simulink model "vehicle_progetto_v1"  (R2022a)
settings: Solver=ode45  StartTime=0.0  StopTime=200.0  MinStep=1e-60  RelTol=1e-3
values from neighbouring files (symbols this model uses):
  a = 2    [vehicle_parameters.m]    (also in vehicle_parameters_v1.m = 1.3; vehicle_parameters_v1_sospensioni.m = 1.3)
  alpha = atan(w/(2*b))    [vehicle_parameters.m]    (also in vehicle_parameters_v1.m; vehicle_parameters_v1_sospensioni.m)
  b = 2.5    [vehicle_parameters.m]    (also in vehicle_parameters_v1.m = 1.8; vehicle_parameters_v1_sospensioni.m = 1.8)
  ca = 0.5    [vehicle_parameters.m]    (also in vehicle_parameters_v1.m; vehicle_parameters_v1_sospensioni.m)
  cs = sqrt(2*ks*M)    [vehicle_parameters.m]    (also in vehicle_parameters_v1.m; vehicle_parameters_v1_sospensioni.m)
  h_gc = 0.15    [vehicle_parameters.m]    (also in vehicle_parameters_v1.m; vehicle_parameters_v1_sospensioni.m = 0.35)
  J_motore = 0.3    [vehicle_parameters_v1.m]    (also in vehicle_parameters_v1_sospensioni.m)
  J_wheel = 0.4    [vehicle_parameters_v1.m]    (also in vehicle_parameters_v1_sospensioni.m)
  Jx = 300    [vehicle_parameters.m]    (also in vehicle_parameters_v1.m; vehicle_parameters_v1_sospensioni.m)
  Jy = 500    [vehicle_parameters.m]    (also in vehicle_parameters_v1.m; vehicle_parameters_v1_sospensioni.m)
  Jz = 600    [vehicle_parameters.m]    (also in vehicle_parameters_v1.m; vehicle_parameters_v1_sospensioni.m)
  K_elettrica_motore = 0.1    [vehicle_parameters_v1.m]    (also in vehicle_parameters_v1_sospensioni.m)
  K_f_motore = 1    [vehicle_parameters_v1.m]    (also in vehicle_parameters_v1_sospensioni.m)
  K_motore = 1    [vehicle_parameters_v1.m]    (also in vehicle_parameters_v1_sospensioni.m)
  k_r = 1e4    (= 10000)    [vehicle_parameters.m]    (also in vehicle_parameters_v1.m = 2000000; vehicle_parameters_v1_sospensioni.m = 2000000)
  k_tu = 1.5e5    (= 150000)    [vehicle_parameters.m]    (also in vehicle_parameters_v1.m = 1500000; vehicle_parameters_v1_sospensioni.m = 1500000)
  k_tv = 4e4    (= 40000)    [vehicle_parameters.m]    (also in vehicle_parameters_v1.m = 400000; vehicle_parameters_v1_sospensioni.m = 400000)
  ks = 40000    [vehicle_parameters.m]    (also in vehicle_parameters_v1.m; vehicle_parameters_v1_sospensioni.m = 9.75)
  L = sqrt(a^2+w^2 /4)    [vehicle_parameters.m]    (also in vehicle_parameters_v1.m; vehicle_parameters_v1_sospensioni.m)
  L_motore = 0.001100    (= 0.0011)    [vehicle_parameters_v1.m]    (also in vehicle_parameters_v1_sospensioni.m)
  M = 1000    [vehicle_parameters.m]    (also in vehicle_parameters_v1.m; vehicle_parameters_v1_sospensioni.m = 1500)
  mu_dyn = 0.4    [vehicle_parameters.m]    (also in vehicle_parameters_v1.m = 0.2; vehicle_parameters_v1_sospensioni.m = 0.2)
  mu_st = 0.8    [vehicle_parameters.m]    (also in vehicle_parameters_v1.m; vehicle_parameters_v1_sospensioni.m)
  r = 0.2    [vehicle_parameters.m]    (also in vehicle_parameters_v1.m = 0.3; vehicle_parameters_v1_sospensioni.m = 0.3)
  R = sqrt(b^2+w^2 /4)    [vehicle_parameters.m]    (also in vehicle_parameters_v1.m; vehicle_parameters_v1_sospensioni.m)
  R_motore = 0.210    (= 0.21)    [vehicle_parameters_v1.m]    (also in vehicle_parameters_v1_sospensioni.m)
  theta = atan(w/(2*a))    [vehicle_parameters.m]    (also in vehicle_parameters_v1.m; vehicle_parameters_v1_sospensioni.m)
  w = 1.6    [vehicle_parameters.m]    (also in vehicle_parameters_v1.m; vehicle_parameters_v1_sospensioni.m)
libraries: simulink x4, slpidlib x1
settings Model: Creator=jackrip  LastModifiedBy=jackrip

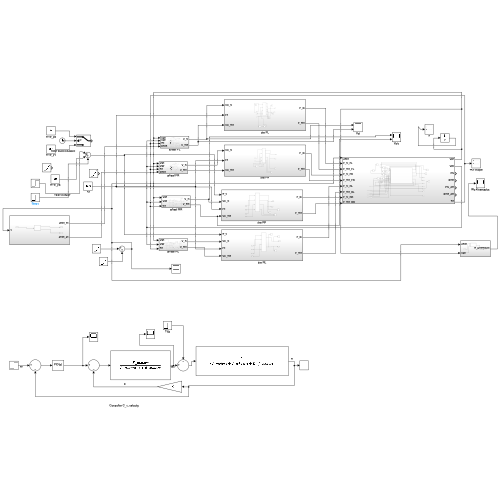
[thumbnail: Simulink's stored preview of the top-level diagram]
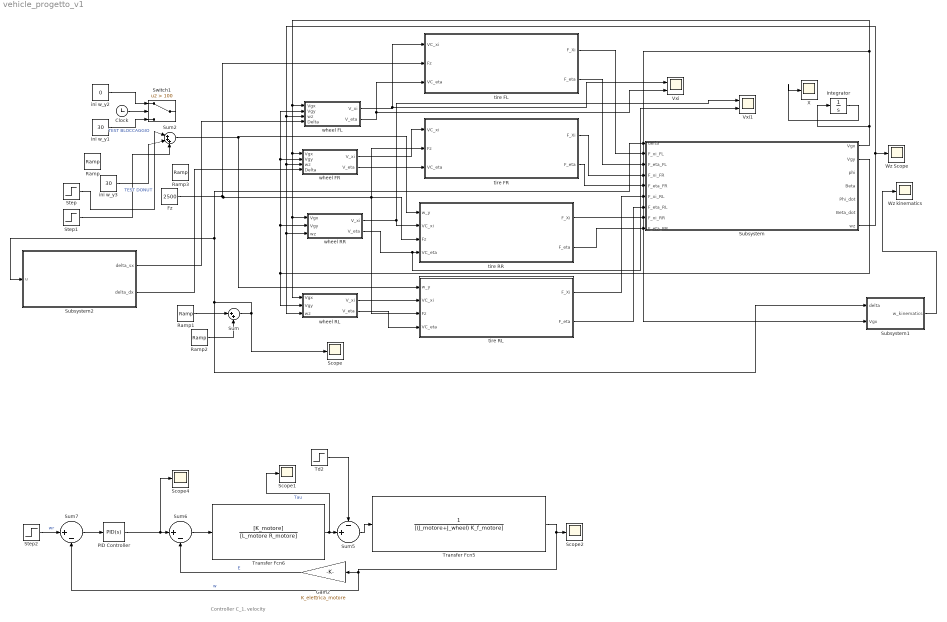
== system vehicle_progetto_v1 ==
  note: Controller C_1, velocity
  " Fz" : Constant  Value=2500
  Clock : Clock
  Gain2 : Gain  Gain=K_elettrica_motore
  Integrator : Integrator
  PID Controller : slpidlib/PID Controller  Controller=PID  Form=Parallel  TimeDomain=Continuous-time  UseExternalTs=off  SampleTime=-1  IntegratorMethod=Forward Euler  FilterMethod=Forward Euler  ControllerParametersSource=internal  P=5  I=1  UseKiTs=off  D=0  N=100  UseFilter=on  TunerSelectOption=Transfer Function Based (PID Tuner App)  InitialConditionSource=internal  InitialConditionForIntegrator=0  InitialConditionForFilter=0  DifferentiatorICPrevScaledInput=0  ExternalReset=none  TrackingMode=off  Kt=1  LimitOutput=off  SatLimitsSource=internal  UpperSaturationLimit=inf  LowerSaturationLimit=-inf  LinearizeAsGain=on  AntiWindupMode=none  Kb=1  POutMin=[]  POutMax=[]  IOutMin=[]  IOutMax=[]  DOutMin=[]  DOutMax=[]  NOutMin=[]  NOutMax=[]  SumOutMin=[]  SumOutMax=[]  SaturationOutMin=[]  SaturationOutMax=[]  PParamMin=[]  PParamMax=[]  IParamMin=[]  IParamMax=[]  DParamMin=[]  DParamMax=[]  NParamMin=[]  NParamMax=[]  KbParamMin=[]  KbParamMax=[]  KtParamMin=[]  KtParamMax=[]  KbOutMin=[]  KbOutMax=[]  KtOutMin=[]  KtOutMax=[]  IntegratorOutMin=[]  IntegratorOutMax=[]  FilterOutMin=[]  FilterOutMax=[]  SumI1OutMin=[]  SumI1OutMax=[]  SumI2OutMin=[]  SumI2OutMax=[]  SumI3OutMin=[]  SumI3OutMax=[]  SumI4OutMin=[]  SumI4OutMax=[]  SumDOutMin=[]  SumDOutMax=[]  DifferentiatorOutMin=[]  DifferentiatorOutMax=[]  FilterDiffOutCoefMin=[]  FilterDiffOutCoefMax=[]  ReciprocalOutMin=[]  ReciprocalOutMax=[]  SumDenOutMin=[]  SumDenOutMax=[]  SumNumOutMin=[]  SumNumOutMax=[]  DivideOutMin=[]  DivideOutMax=[]  UdiffTsProdOutMin=[]  UdiffTsProdOutMax=[]  NTsProdOutMin=[]  NTsProdOutMax=[]  UintegralTsProdOutMin=[]  UintegralTsProdOutMax=[]  UngainTsProdOutMin=[]  UngainTsProdOutMax=[]  IntegratorContinuousStateAttributes=''  IntegratorStateMustResolveToSignalObject=off  IntegratorRTWStateStorageClass=Auto  FilterContinuousStateAttributes=''  FilterStateMustResolveToSignalObject=off  FilterRTWStateStorageClass=Auto  ParallelPVariant=InternalParameters  IdealPVariant=Disabled  IVariant=InternalParameters  DVariant=InternalParameters  IntegratorVariant=Continuous  SatVariant=Disabled  AWVariant=Passthrough  PCopyVariant=Disabled  TRVariant=Disabled  FdbkBlocksVariant=Forward  IdealPFdbkVariant=Disabled  SatFdbkVariant=Disabled  DerivativeFilterVariant=ContFilter  NVariant=InternalParameters  NCopyVariant=Disabled  FilterICVariant=InternalICsFilter  IntegratorICVariant=InternalICs  ExternalResetVariant=Disabled  TRSumVariant=Passthrough  SumFdbkVariant=Disabled  SumVariant=Sum_PID  TsampFilterVariant=InternalTs  TsampNgainVariant=Passthrough  TsampIntegralVariant=Passthrough  ExternalSaturationOutDataTypeStr=Inherit: Same as second input  aMode=0
  Ramp : simulink/Sources/Ramp  slope=0  start=100  InitialOutput=0
  Ramp1 : simulink/Sources/Ramp  slope=-0.3  start=50  InitialOutput=0
  Ramp2 : simulink/Sources/Ramp  slope=+0.3  start=51  InitialOutput=0
  Ramp3 : simulink/Sources/Ramp  slope=0  start=103  InitialOutput=0
  Scope{,1..2,4} (4 alike) : Scope
  Step : Step  Time=100  After=25*0  SampleTime=0
  Step1 : Step  Time=101.5  After=-25*0  SampleTime=0
  Step2 : Step  Time=0  After=30  SampleTime=0
  Subsystem : Subsystem
  Subsystem1 : Subsystem
  Subsystem2 : Subsystem
  Sum : Sum  Inputs=|++
  Sum2 : Sum  Inputs=|+++
  Sum5 : Sum  Inputs=-+|
  Sum6 : Sum  Inputs=|+-
  Sum7 : Sum  Inputs=|+-
  Switch1 : Switch  Criteria=u2 > Threshold  Threshold=100  SaturateOnIntegerOverflow=off  InputSameDT=off
  Td2 : Step  Time=3  After=0.4*0  SampleTime=0
  Transfer Fcn5 : TransferFcn  Denominator=[(J_motore+J_wheel) K_f_motore]
  Transfer Fcn6 : TransferFcn  Numerator=[K_motore]  Denominator=[L_motore R_motore]
  Vxi : Scope  NumInputPorts=2
  Vxi1 : Scope  NumInputPorts=2
  Wz Scope : Scope
  Wz kinematics : Scope
  X : Scope
  ini w_y1 : Constant  Value=30
  ini w_y2 : Constant  Value=0
  ini w_y3 : Constant  Value=30
  tire FL : Subsystem
  tire FR : Subsystem
  tire RL : Subsystem
  tire RR : Subsystem
  wheel FL : Subsystem
  wheel FR : Subsystem
  wheel RL : Subsystem
  wheel RR : Subsystem
  wires:
  wheel FL/1(V_xi) -> Vxi/1, tire FL/1(VC_xi)
  wheel FL/2(V_eta) -> Vxi/2, tire FL/3(VC_eta)
  tire FL/1(F_Xi) -> Subsystem/2(F_xi_FL)
  tire FL/2(F_eta) -> Subsystem/3(F_eta_FL)
  tire RL/1(F_Xi) -> Subsystem/6(F_xi_RL)
  tire RL/2(F_eta) -> Subsystem/7(F_eta_RL)
  tire RR/1(F_Xi) -> Subsystem/8(F_xi_RR)
  tire RR/2(F_eta) -> Subsystem/9(F_eta_RR)
  tire FR/1(F_Xi) -> Subsystem/4(F_xi_FR)
  tire FR/2(F_eta) -> Subsystem/5(F_eta_FR)
  wheel FR/1(V_xi) -> tire FR/1(VC_xi)
  wheel FR/2(V_eta) -> tire FR/3(VC_eta)
  wheel RL/1(V_xi) -> tire RL/2(VC_xi)
  wheel RR/1(V_xi) -> Vxi1/1, tire RR/2(VC_xi)
  wheel RR/2(V_eta) -> Vxi1/2, tire RR/4(VC_eta)
  wheel RL/2(V_eta) -> tire RL/4(VC_eta)
  Subsystem/1(Vgx) -> wheel RL/1(Vgx), wheel RR/1(Vgx), wheel FR/1(Vgx), wheel FL/1(Vgx), Subsystem1/2(Vgx), Integrator/1
  Subsystem/2(Vgy) -> wheel FL/2(Vgy), wheel FR/2(Vgy), wheel RR/2(Vgy), wheel RL/2(Vgy)
  Subsystem/7(wz) -> Wz Scope/1, wheel RL/3(wz), wheel RR/3(wz), wheel FR/3(wz), wheel FL/3(wz)
  Sum2/1 -> tire RR/1(w_y), tire RL/1(w_y)
  " Fz"/1 -> tire RL/3(Fz), tire FR/2(Fz), tire RR/3(Fz), tire FL/2(Fz)
  Ramp2/1 -> Sum/2
  Ramp1/1 -> Sum/1
  Integrator/1 -> X/1
  Clock/1 -> Switch1/2
  ini w_y1/1 -> Switch1/3  "TEST BLOCCAGGIO"
  ini w_y2/1 -> Switch1/1
  ini w_y3/1 -> Sum2/2
  Transfer Fcn5/1 -> Gain2/1, Sum7/2, Scope2/1  "w"
  Sum5/1 -> Transfer Fcn5/1
  Gain2/1 -> Sum6/2  "E"
  Td2/1 -> Sum5/1
  Sum6/1 -> Transfer Fcn6/1
  Transfer Fcn6/1 -> Scope1/1, Sum5/2  "Tau"
  Sum7/1 -> PID Controller/1
  Step2/1 -> Sum7/1  "wr"
  PID Controller/1 -> Sum6/1, Scope4/1
  Sum/1 -> Scope/1, Subsystem2/1(u), Subsystem/1(delta), Subsystem1/1(delta)
  Step/1 -> Sum2/1  "TEST DONUT"
  Step1/1 -> Sum2/3
  Subsystem1/1(w_kinematics) -> Wz kinematics/1
  Subsystem2/1(delta_sx) -> wheel FL/4(Delta)
  Subsystem2/2(delta_dx) -> wheel FR/4(Delta)

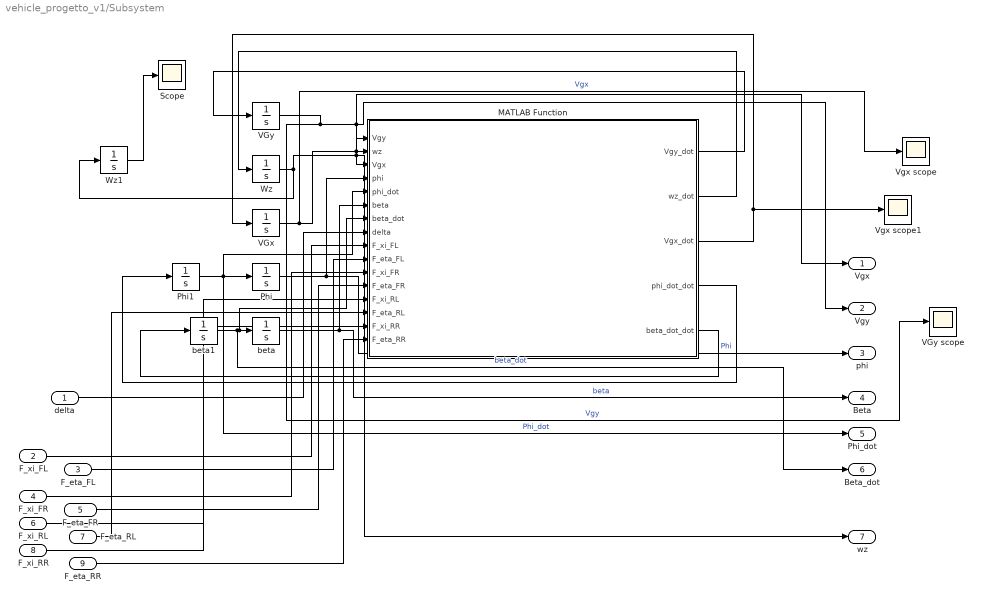
== system vehicle_progetto_v1/Subsystem ==
  delta : Inport
  F_xi_FL : Inport  Port=2
  F_eta_FL : Inport  Port=3
  F_xi_FR : Inport  Port=4
  F_eta_FR : Inport  Port=5
  F_xi_RL : Inport  Port=6
  F_eta_RL : Inport  Port=7
  F_xi_RR : Inport  Port=8
  F_eta_RR : Inport  Port=9
  " VGy scope" : Scope
  MATLAB Function : MATLAB Function  TreatAsAtomicUnit=on
  Phi : Integrator
  Phi1 : Integrator
  Scope : Scope
  VGx : Integrator  InitialCondition=0.055
  VGy : Integrator
  Vgx scope : Scope
  Vgx scope1 : Scope
  Wz : Integrator
  Wz1 : Integrator
  beta : Integrator
  beta1 : Integrator
  Vgx : Outport
  Vgy : Outport  Port=2
  phi : Outport  Port=3
  Beta : Outport  Port=4
  Phi_dot : Outport  Port=5
  Beta_dot : Outport  Port=6
  wz : Outport  Port=7
  wires:
  Phi1/1 -> Phi_dot/1, MATLAB Function/5(phi_dot), Phi/1  "Phi_dot"
  VGy/1 -> Vgy/1, MATLAB Function/1(Vgy), " VGy scope"/1  "Vgy"
  MATLAB Function/2(wz_dot) -> Wz/1
  Wz/1 -> Wz1/1, wz/1, MATLAB Function/2(wz)
  MATLAB Function/3(Vgx_dot) -> VGx/1, Vgx scope1/1
  VGx/1 -> Vgx scope/1, Vgx/1, MATLAB Function/3(Vgx)  "Vgx"
  MATLAB Function/4(phi_dot_dot) -> Phi1/1
  Phi/1 -> phi/1, MATLAB Function/4(phi)  "Phi"
  beta1/1 -> MATLAB Function/7(beta_dot), beta/1, Beta_dot/1  "beta_dot"
  MATLAB Function/5(beta_dot_dot) -> beta1/1
  beta/1 -> Beta/1, MATLAB Function/6(beta)  "beta"
  delta/1 -> MATLAB Function/8(delta)
  F_xi_FL/1 -> MATLAB Function/9(F_xi_FL)
  F_eta_FL/1 -> MATLAB Function/10(F_eta_FL)
  F_xi_FR/1 -> MATLAB Function/11(F_xi_FR)
  F_eta_FR/1 -> MATLAB Function/12(F_eta_FR)
  F_xi_RL/1 -> MATLAB Function/13(F_xi_RL)
  F_eta_RL/1 -> MATLAB Function/14(F_eta_RL)
  F_xi_RR/1 -> MATLAB Function/15(F_xi_RR)
  F_eta_RR/1 -> MATLAB Function/16(F_eta_RR)
  Wz1/1 -> Scope/1
  MATLAB Function/1(Vgy_dot) -> VGy/1

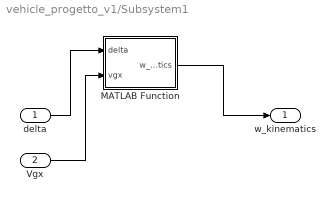
== system vehicle_progetto_v1/Subsystem1 ==
  delta : Inport
  Vgx : Inport  Port=2
  MATLAB Function : MATLAB Function  TreatAsAtomicUnit=on
  w_kinematics : Outport
  wires:
  Vgx/1 -> MATLAB Function/2(vgx)
  delta/1 -> MATLAB Function/1(delta)
  MATLAB Function/1(w_kinematics) -> w_kinematics/1

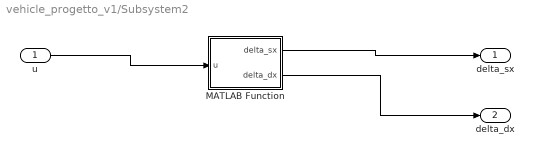
== system vehicle_progetto_v1/Subsystem2 ==
  u : Inport
  MATLAB Function : MATLAB Function  TreatAsAtomicUnit=on
  delta_sx : Outport
  delta_dx : Outport  Port=2
  wires:
  u/1 -> MATLAB Function/1(u)
  MATLAB Function/1(delta_sx) -> delta_sx/1
  MATLAB Function/2(delta_dx) -> delta_dx/1

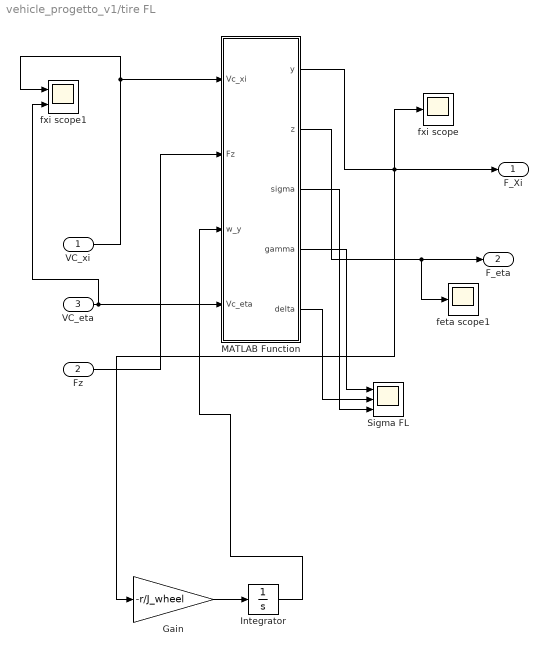
== system vehicle_progetto_v1/tire FL ==
  VC_xi : Inport
  Fz : Inport  Port=2
  VC_eta : Inport  Port=3
  Gain : Gain  Gain=-r/J_wheel
  Integrator : Integrator  InitialCondition=0.0001
  MATLAB Function : MATLAB Function  TreatAsAtomicUnit=on
  Sigma FL : Scope  NumInputPorts=3
  feta scope1 : Scope
  fxi scope : Scope
  fxi scope1 : Scope  NumInputPorts=2
  F_Xi : Outport
  F_eta : Outport  Port=2
  wires:
  MATLAB Function/1(y) -> Gain/1, F_Xi/1, fxi scope/1
  MATLAB Function/2(z) -> feta scope1/1, F_eta/1
  VC_eta/1 -> fxi scope1/2, MATLAB Function/4(Vc_eta)
  MATLAB Function/3(sigma) -> Sigma FL/3
  MATLAB Function/4(gamma) -> Sigma FL/1
  MATLAB Function/5(delta) -> Sigma FL/2
  Gain/1 -> Integrator/1
  VC_xi/1 -> fxi scope1/1, MATLAB Function/1(Vc_xi)
  Integrator/1 -> MATLAB Function/3(w_y)
  Fz/1 -> MATLAB Function/2(Fz)

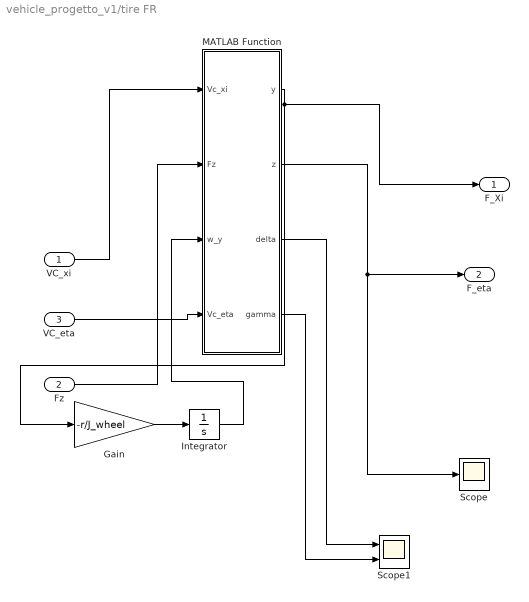
== system vehicle_progetto_v1/tire FR ==
  VC_xi : Inport
  Fz : Inport  Port=2
  VC_eta : Inport  Port=3
  Gain : Gain  Gain=-r/J_wheel
  Integrator : Integrator  InitialCondition=0.00001
  MATLAB Function : MATLAB Function  TreatAsAtomicUnit=on
  Scope : Scope
  Scope1 : Scope  NumInputPorts=2
  F_Xi : Outport
  F_eta : Outport  Port=2
  wires:
  MATLAB Function/1(y) -> Gain/1, F_Xi/1
  VC_xi/1 -> MATLAB Function/1(Vc_xi)
  MATLAB Function/2(z) -> Scope/1, F_eta/1
  VC_eta/1 -> MATLAB Function/4(Vc_eta)
  MATLAB Function/3(delta) -> Scope1/1
  Gain/1 -> Integrator/1
  Integrator/1 -> MATLAB Function/3(w_y)
  MATLAB Function/4(gamma) -> Scope1/2
  Fz/1 -> MATLAB Function/2(Fz)

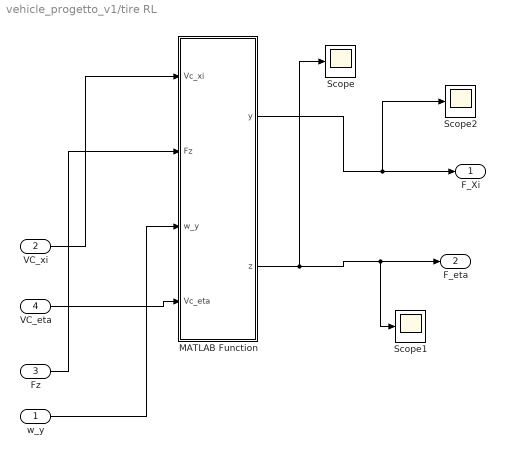
== system vehicle_progetto_v1/tire RL ==
  w_y : Inport
  VC_xi : Inport  Port=2
      settings: AttributesFormatString=|
      | Velocità Del centro della ruota diretta lungo l'asse della ruota
      | Se la macchina stesse andando dritta sarebbe uguale a vgx
  Fz : Inport  Port=3
  VC_eta : Inport  Port=4
  MATLAB Function : MATLAB Function  TreatAsAtomicUnit=on
  Scope : Scope
  Scope1 : Scope
  Scope2 : Scope
  F_Xi : Outport
  F_eta : Outport  Port=2
  wires:
  MATLAB Function/1(y) -> Scope2/1, F_Xi/1
  VC_xi/1 -> MATLAB Function/1(Vc_xi)
  w_y/1 -> MATLAB Function/3(w_y)
  MATLAB Function/2(z) -> Scope/1, Scope1/1, F_eta/1
  VC_eta/1 -> MATLAB Function/4(Vc_eta)
  Fz/1 -> MATLAB Function/2(Fz)

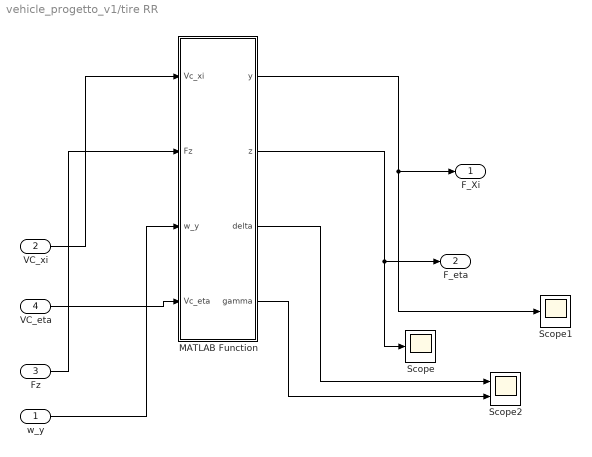
== system vehicle_progetto_v1/tire RR ==
  w_y : Inport
  VC_xi : Inport  Port=2
  Fz : Inport  Port=3
  VC_eta : Inport  Port=4
  MATLAB Function : MATLAB Function  TreatAsAtomicUnit=on
  Scope : Scope
  Scope1 : Scope
  Scope2 : Scope  NumInputPorts=2
  F_Xi : Outport
  F_eta : Outport  Port=2
  wires:
  MATLAB Function/1(y) -> Scope1/1, F_Xi/1
  VC_xi/1 -> MATLAB Function/1(Vc_xi)
  w_y/1 -> MATLAB Function/3(w_y)
  MATLAB Function/2(z) -> Scope/1, F_eta/1
  VC_eta/1 -> MATLAB Function/4(Vc_eta)
  MATLAB Function/3(delta) -> Scope2/1
  MATLAB Function/4(gamma) -> Scope2/2
  Fz/1 -> MATLAB Function/2(Fz)

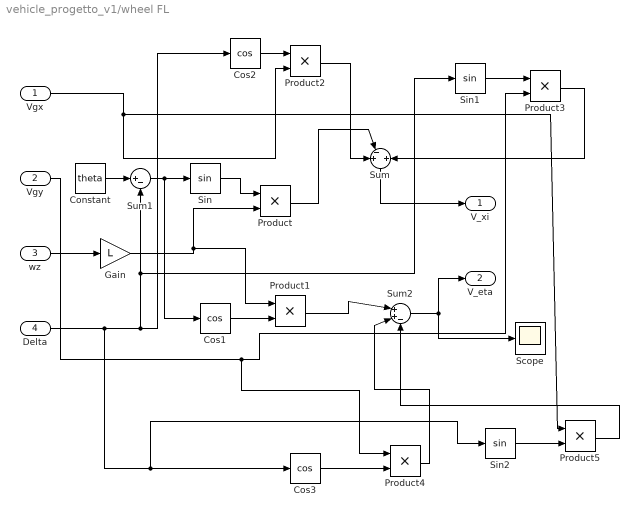
== system vehicle_progetto_v1/wheel FL ==
  Vgx : Inport
  Vgy : Inport  Port=2
  wz : Inport  Port=3
  Delta : Inport  Port=4
  Constant : Constant  Value=theta
  Cos1 : Trigonometry  Operator=cos
  Cos2 : Trigonometry  Operator=cos
  Cos3 : Trigonometry  Operator=cos
  Gain : Gain  Gain=L
  Product{,1..5} (6 alike) : Product
  Scope : Scope
  Sin : Trigonometry
  Sin1 : Trigonometry
  Sin2 : Trigonometry
  Sum : Sum  Inputs=+-|+
  Sum1 : Sum  Inputs=|+-
  Sum2 : Sum  Inputs=|++-
  V_xi : Outport
  V_eta : Outport  Port=2
  wires:
  Vgx/1 -> Product5/1, Product2/2
  wz/1 -> Gain/1
  Sin/1 -> Product/1
  Constant/1 -> Sum1/1
  Sum1/1 -> Cos1/1, Sin/1
  Delta/1 -> Sin2/1, Cos3/1, Sum1/2, Sin1/1, Cos2/1
  Product/1 -> Sum/2
  Sum/1 -> V_xi/1
  Cos1/1 -> Product1/2
  Gain/1 -> Product/2, Product1/1
  Product1/1 -> Sum2/1
  Sum2/1 -> Scope/1, V_eta/1
  Vgy/1 -> Product4/1, Product3/2
  Cos2/1 -> Product2/1
  Product2/1 -> Sum/1
  Sin1/1 -> Product3/1
  Product3/1 -> Sum/3
  Cos3/1 -> Product4/2
  Product4/1 -> Sum2/2
  Sin2/1 -> Product5/2
  Product5/1 -> Sum2/3

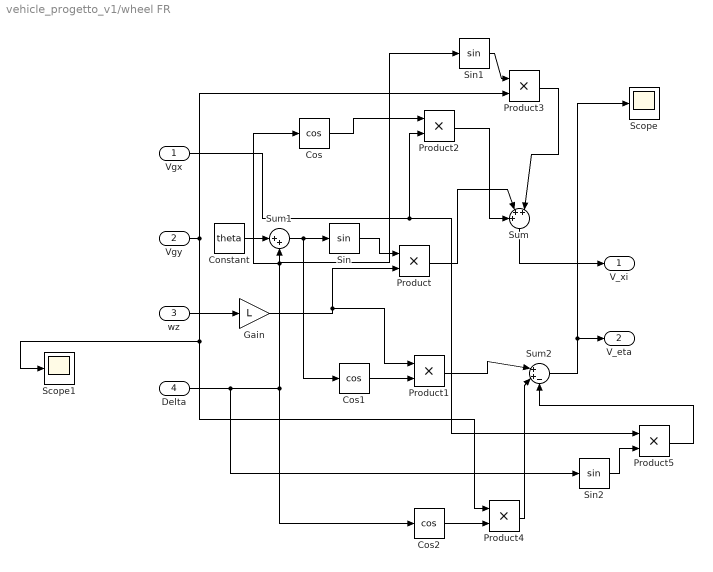
== system vehicle_progetto_v1/wheel FR ==
  Vgx : Inport
  Vgy : Inport  Port=2
  wz : Inport  Port=3
  Delta : Inport  Port=4
  Constant : Constant  Value=theta
  Cos : Trigonometry  Operator=cos
  Cos1 : Trigonometry  Operator=cos
  Cos2 : Trigonometry  Operator=cos
  Gain : Gain  Gain=L
  Product{,1..5} (6 alike) : Product
  Scope : Scope
  Scope1 : Scope
  Sin : Trigonometry
  Sin1 : Trigonometry
  Sin2 : Trigonometry
  Sum : Sum  Inputs=+++|
  Sum1 : Sum  Inputs=|++
  Sum2 : Sum  Inputs=|++-
  V_xi : Outport
  V_eta : Outport  Port=2
  wires:
  Vgx/1 -> Product5/1, Product2/2
  wz/1 -> Gain/1
  Sin/1 -> Product/1
  Constant/1 -> Sum1/1
  Sum1/1 -> Cos1/1, Sin/1
  Delta/1 -> Sin2/1, Cos2/1, Cos/1, Sum1/2, Sin1/1
  Product/1 -> Sum/2
  Sum/1 -> V_xi/1
  Cos1/1 -> Product1/2
  Gain/1 -> Product/2, Product1/1
  Product1/1 -> Sum2/1
  Sum2/1 -> Scope/1, V_eta/1
  Vgy/1 -> Product4/1, Scope1/1, Product3/2
  Cos/1 -> Product2/1
  Product2/1 -> Sum/1
  Sin1/1 -> Product3/1
  Product3/1 -> Sum/3
  Cos2/1 -> Product4/2
  Product4/1 -> Sum2/2
  Sin2/1 -> Product5/2
  Product5/1 -> Sum2/3

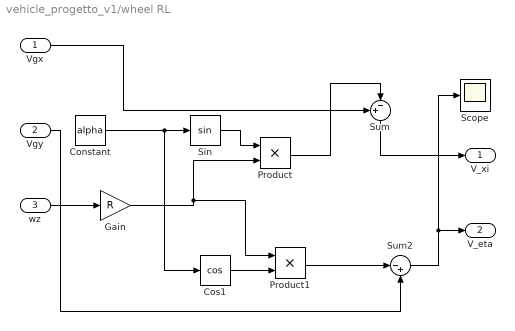
== system vehicle_progetto_v1/wheel RL ==
  Vgx : Inport
  Vgy : Inport  Port=2
  wz : Inport  Port=3
  Constant : Constant  Value=alpha
  Cos1 : Trigonometry  Operator=cos
  Gain : Gain  Gain=R
  Product : Product
  Product1 : Product
  Scope : Scope
  Sin : Trigonometry
  Sum : Sum  Inputs=+-|
  Sum2 : Sum  Inputs=|-+
  V_xi : Outport
  V_eta : Outport  Port=2
  wires:
  Vgx/1 -> Sum/1
  wz/1 -> Gain/1
  Sin/1 -> Product/1
  Constant/1 -> Cos1/1, Sin/1
  Product/1 -> Sum/2
  Sum/1 -> V_xi/1
  Cos1/1 -> Product1/2
  Gain/1 -> Product/2, Product1/1
  Product1/1 -> Sum2/1
  Sum2/1 -> Scope/1, V_eta/1
  Vgy/1 -> Sum2/2

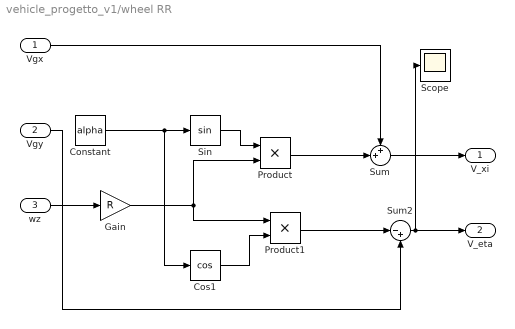
== system vehicle_progetto_v1/wheel RR ==
  Vgx : Inport
  Vgy : Inport  Port=2
  wz : Inport  Port=3
  Constant : Constant  Value=alpha
  Cos1 : Trigonometry  Operator=cos
  Gain : Gain  Gain=R
  Product : Product
  Product1 : Product
  Scope : Scope
  Sin : Trigonometry
  Sum : Sum  Inputs=++|
  Sum2 : Sum  Inputs=|-+
  V_xi : Outport
  V_eta : Outport  Port=2
  wires:
  Vgx/1 -> Sum/1
  wz/1 -> Gain/1
  Sin/1 -> Product/1
  Constant/1 -> Cos1/1, Sin/1
  Product/1 -> Sum/2
  Sum/1 -> V_xi/1
  Cos1/1 -> Product1/2
  Gain/1 -> Product/2, Product1/1
  Product1/1 -> Sum2/1
  Sum2/1 -> Scope/1, V_eta/1
  Vgy/1 -> Sum2/2

== matlab function vehicle_progetto_v1/tire RR/MATLAB Function ==
  data: Vc_xi input; y output; Fz input; w_y input; r parameter; mu_st parameter; k_r parameter; mu_dyn parameter; k_tv parameter; k_tu parameter; z output; Vc_eta input; delta output; gamma output
function [y,z,delta, gamma] = fcn(Vc_xi, Fz, w_y,r, mu_st, k_r, mu_dyn, k_tv, k_tu, Vc_eta)
c = (Fz*r*12/(k_r*0.2))^(1/3);
S = c*0.2;
sigma=(Vc_xi-w_y*r)/Vc_xi;
gamma = Vc_eta/Vc_xi;
delta = r*2*sqrt(k_tu^2*sigma^2+k_tv^2*gamma^2)/(c*mu_st*k_r);
if delta>1
    delta=1;
end
F_xi = -sign(Vc_xi-w_y*r)*mu_st*Fz*(6*abs(sigma)/(sqrt(sigma^2+gamma^2))*mu_dyn/mu_st*(0.5-1/3*delta)*(delta)^2+S*k_tu*c/(2*mu_st*Fz)*(delta-1)^2*abs(sigma));
F_eta = -sign(Vc_eta)*abs(mu_st*Fz*(6*gamma/(sqrt(sigma^2+gamma^2))*mu_dyn/mu_st*(0.5-1/3*delta)*(delta)^2+S*k_tv*c/(2*mu_st*Fz)*(delta-1)^2*gamma));
y = F_xi;
z = F_eta;

== matlab function vehicle_progetto_v1/tire FR/MATLAB Function ==
  data: Vc_xi input; y output; Fz input; w_y input; r parameter; mu_st parameter; k_r parameter; mu_dyn parameter; k_tv parameter; k_tu parameter; z output; Vc_eta input; delta output; gamma output
function [y,z, delta, gamma] = fcn(Vc_xi, Fz, w_y,r, mu_st, k_r, mu_dyn, k_tv, k_tu, Vc_eta)
c = (Fz*r*12/(k_r*0.2))^(1/3);
S = c*0.2;
sigma=(Vc_xi-w_y*r)/Vc_xi;
gamma = Vc_eta/Vc_xi;
delta = r*2*sqrt(k_tu^2*sigma^2+k_tv^2*gamma^2)/(c*mu_st*k_r);
if delta>1
    delta=1;
end
F_xi = -sign(Vc_xi-w_y*r)*mu_st*Fz*(6*abs(sigma)/(sqrt(sigma^2+gamma^2))*mu_dyn/mu_st*(0.5-1/3*delta)*(delta)^2+S*k_tu*c/(2*mu_st*Fz)*(delta-1)^2*abs(sigma));
F_eta = -sign(Vc_eta)*abs(mu_st*Fz*(6*gamma/(sqrt(sigma^2+gamma^2))*mu_dyn/mu_st*(0.5-1/3*delta)*(delta)^2+S*k_tv*c/(2*mu_st*Fz)*(delta-1)^2*gamma));
y = F_xi;
z = F_eta;

== matlab function vehicle_progetto_v1/Subsystem1/MATLAB Function ==
  data: delta input; w_kinematics output; vgx input; a parameter; b parameter
function w_kinematics = fcn(delta, vgx, a, b)
beta = atan(b*tan(delta)/(a+b))
w_kinematics = vgx*tan(delta)*cos(beta)/(a+b);

== matlab function vehicle_progetto_v1/Subsystem2/MATLAB Function ==
  data: u input; delta_sx output; delta_dx output; a parameter; b parameter; w parameter
function [delta_sx,delta_dx]= fcn(u, a, b, w)
delta_sx = atan(2*(a+b)*sin(u)/(2*(a+b)*cos(u)-w*sin(u)));
delta_dx = atan(2*(a+b)*sin(u)/(2*(a+b)*cos(u)+w*sin(u)));
y = u;

== matlab function vehicle_progetto_v1/tire RL/MATLAB Function ==
  data: Vc_xi input; y output; Fz input; w_y input; r parameter; mu_st parameter; k_r parameter; mu_dyn parameter; k_tv parameter; k_tu parameter; z output; Vc_eta input
function [y,z] = fcn(Vc_xi, Fz, w_y,r, mu_st, k_r, mu_dyn, k_tv, k_tu, Vc_eta)
c = (Fz*r*12/(k_r*0.2))^(1/3);
S = c*0.2;
sigma=(Vc_xi-w_y*r)/Vc_xi;
gamma = Vc_eta/Vc_xi;
delta = r*2*sqrt(k_tu^2*sigma^2+k_tv^2*gamma^2)/(c*mu_st*k_r);
if delta>1
    delta=1;
end
F_xi = -sign(Vc_xi-w_y*r)*mu_st*Fz*(6*abs(sigma)/(sqrt(sigma^2+gamma^2))*mu_dyn/mu_st*(0.5-1/3*delta)*(delta)^2+S*k_tu*c/(2*mu_st*Fz)*(delta-1)^2*abs(sigma));
F_eta = -sign(Vc_eta)*abs(mu_st*Fz*(6*gamma/(sqrt(sigma^2+gamma^2))*mu_dyn/mu_st*(0.5-1/3*delta)*(delta)^2+S*k_tv*c/(2*mu_st*Fz)*(delta-1)^2*gamma));
y = F_xi;
z = F_eta;

== matlab function vehicle_progetto_v1/tire FL/MATLAB Function ==
  data: Vc_xi input; y output; Fz input; w_y input; r parameter; mu_st parameter; k_r parameter; mu_dyn parameter; k_tv parameter; k_tu parameter; z output; Vc_eta input; sigma output; gamma output; delta output
function [y,z,sigma,gamma,delta] = fcn(Vc_xi, Fz, w_y,r, mu_st, k_r, mu_dyn, k_tv, k_tu, Vc_eta)
c = (Fz*r*12/(k_r*0.2))^(1/3);
S = c*0.2;
sigma=(Vc_xi-w_y*r)/Vc_xi;
gamma = Vc_eta/Vc_xi;
delta = r*2*sqrt(k_tu^2*sigma^2+k_tv^2*gamma^2)/(c*mu_st*k_r);
if delta>1
    delta=1;
end
F_xi = -sign(Vc_xi-w_y*r)*mu_st*Fz*(6*abs(sigma)/(sqrt(sigma^2+gamma^2))*mu_dyn/mu_st*(0.5-1/3*delta)*(delta)^2+S*k_tu*c/(2*mu_st*Fz)*(delta-1)^2*abs(sigma));
F_eta = -sign(Vc_eta)*abs(mu_st*Fz*(6*gamma/(sqrt(sigma^2+gamma^2))*mu_dyn/mu_st*(0.5-1/3*delta)*(delta)^2+S*k_tv*c/(2*mu_st*Fz)*(delta-1)^2*gamma));
y = F_xi;
z = F_eta;

== matlab function vehicle_progetto_v1/Subsystem/MATLAB Function ==
  data: Vgy input; Vgy_dot output; wz input; Vgx input; phi input; phi_dot input; beta input; beta_dot input; delta input; F_xi_FL input; F_eta_FL input; F_xi_FR input; F_eta_FR input; F_xi_RL input; F_eta_RL input; F_xi_RR input; F_eta_RR input; wz_dot output; Vgx_dot output; phi_dot_dot output; beta_dot_dot output; M parameter; a parameter; b parameter; h_gc parameter; Jx parameter; Jy parameter; Jz parameter; ks parameter; cs parameter; ca parameter
function [Vgy_dot, wz_dot, Vgx_dot, phi_dot_dot, beta_dot_dot] = fcn(Vgy, wz, Vgx, phi, phi_dot, beta, beta_dot, delta, F_xi_FL, F_eta_FL,  F_xi_FR, F_eta_FR,  F_xi_RL, F_eta_RL, F_xi_RR, F_eta_RR, M, a, b, h_gc, Jx, Jy, Jz, ks, cs,ca)

F_air=ca*Vgx^2;
Fy = (F_eta_RL + F_eta_RR)+ (F_eta_FL + F_eta_FR)*cos(delta) + (F_xi_FL + F_xi_FR)*sin(delta); %data dalla trazione delle ruote

% disp(F_eta_RL)
% disp(F_eta_RR)
% disp(F_eta_FR)
% disp(F_xi_FL)
% disp(F_xi_FR)
% disp(Fy)
% disp(M)
% disp(wz)
% disp(Vgx)

Vgy_dot = Fy/M - wz*Vgx ;
% disp(Vgy_dot)

Mgz = -(F_eta_RL + F_eta_RR)*b+(F_eta_FL + F_eta_FR)*cos(delta)*a+(F_xi_FL + F_xi_FR)*sin(delta)*a;
wz_dot = Mgz/Jz;
Fx = (F_xi_RL + F_xi_RR)+(F_xi_FL + F_xi_FR)*cos(delta)-(F_eta_FL + F_eta_FR)*sin(delta);
Vgx_dot = Fx/M -F_air/M*sign(Vgx);
phi_dot_dot = -ks*phi/Jx -cs*phi_dot/Jx + Fy*h_gc/Jx;
My = Fx*h_gc;
beta_dot_dot = -ks*beta/Jy -cs*beta_dot/Jy + My/Jy;
